simulink model "PM_fnc20_abs_ampslimit_1Dlookup_TestHarness_backup"  (R2022a)
settings: Solver=VariableStepAuto  StartTime=0.0  StopTime=inf  RelTol=1e-3
settings Model: Creator=306427  LastModifiedBy=306427

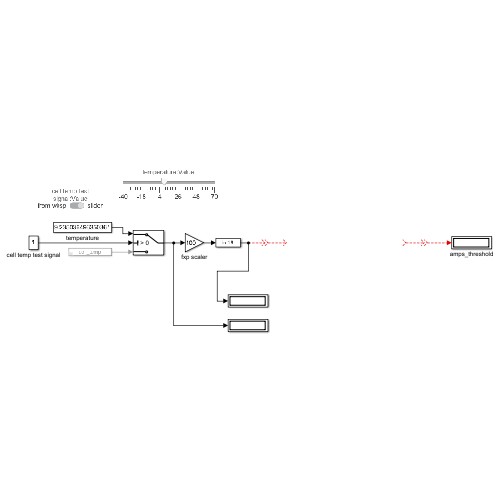
[thumbnail: Simulink's stored preview of the top-level diagram]
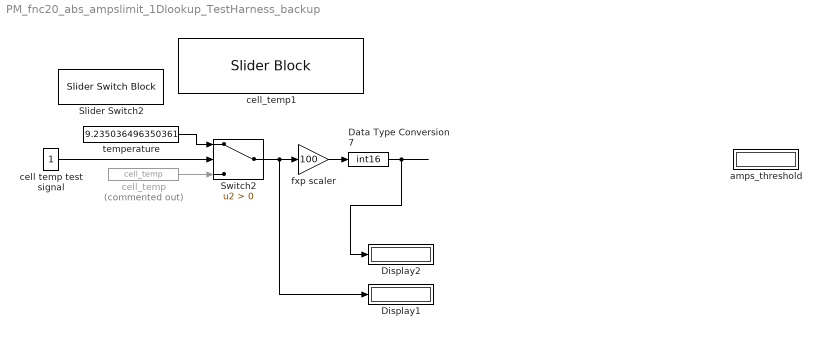
== system PM_fnc20_abs_ampslimit_1Dlookup_TestHarness_backup ==
  Data Type Conversion7 : DataTypeConversion  OutDataTypeStr=int16  SaturateOnIntegerOverflow=off  RndMeth=Floor
  Display1 : Display
  Display2 : Display
  Slider Switch2 : SliderSwitchBlock
      settings: Values={{'from wksp', 'slider'}, [0 1]}
  Switch2 : Switch  Criteria=u2 > Threshold  SaturateOnIntegerOverflow=off  InputSameDT=off
  amps_threshold : Display
  cell temp test signal : Constant
  cell_temp : FromWorkspace  Commented=on  VariableName=cell_temp  OutDataTypeStr=double  SampleTime=[0, 1]
  cell_temp1 : SliderBlock  ScaleMin=-40  ScaleMax=70
  fxp scaler : Gain  Gain=100
  temperature : Constant  Value=9.235036496350361  OutDataTypeStr=double
  wires:
  ? -> ?
  ? -> ?
  temperature/1 -> Switch2/1
  cell_temp/1 -> Switch2/3
  ? -> amps_threshold/1
  cell temp test signal/1 -> Switch2/2
  Switch2/1 -> Display1/1, fxp scaler/1
  Data Type Conversion7/1 -> Display2/1
  fxp scaler/1 -> Data Type Conversion7/1
